simulink model "wind_pmsm_inv_dcBus"  (R2016a)
settings: Solver=VariableStepAuto  StartTime=0.0  StopTime=0.25*100e6  RelTol=1e-3
libraries: xbsIndex_r4 x34, powerlib_meascontrol x2
settings Model: Creator=Jorge  LastModifiedBy=Jorge

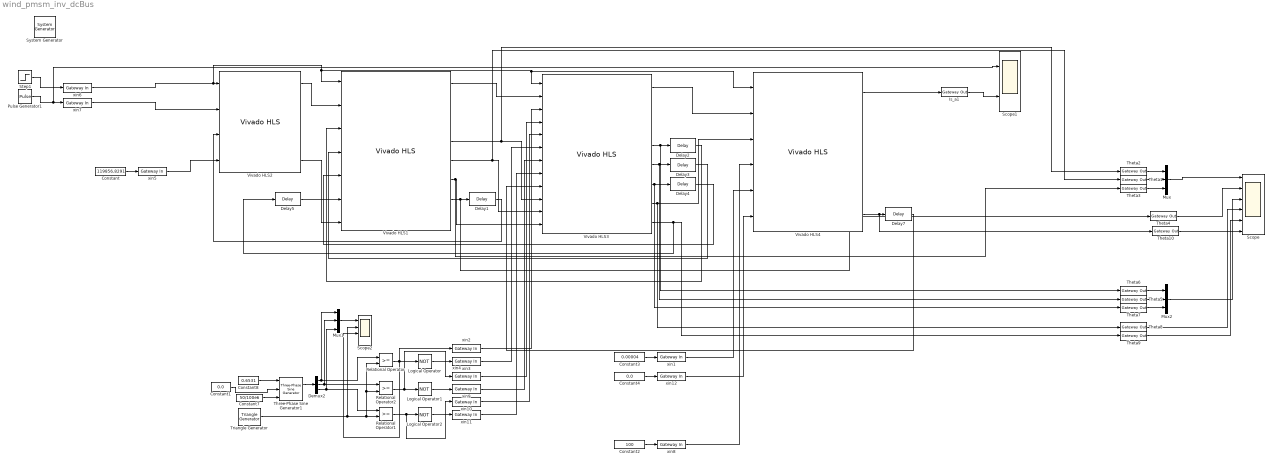
== system wind_pmsm_inv_dcBus ==
  " System Generator" : xbsIndex_r4/ System Generator  Tag=genX  xilinxfamily=zynq  part=xc7z020  speed=-1  package=clg400  synthesis_tool=Vivado  clock_wrapper=Clock Enables  directory=./netlist  proj_type=Vivado  Synth_file=Vivado Synthesis Defaults  Impl_file=Vivado Implementation Defaults  testbench=off  simulink_period=1  sysclk_period=10  dcm_input_clock_period=10  incr_netlist=off  trim_vbits=Everywhere in SubSystem  dbl_ovrd=According to Block Masks  core_generation=According to Block Masks  run_coregen=off  deprecated_control=off  eval_field=0  block_type=sysgen
  Constant : Constant  Value=119856.8291
  Constant1 : Constant  Value=0.0
  Constant2 : Constant  Value=100
  Constant3 : Constant  Value=0.00004
  Constant4 : Constant  Value=0.0
  Constant7 : Constant  Value=50/100e6
  Constant8 : Constant  Value=0.6531
  Delay{1..5,7} (6 alike) : xbsIndex_r4/Delay  rst=off  infoeditControl=Selection of Reset will increase slice count due to use of real FFs and instead of SRLs  en=off  latency=1  reg_retiming=off  dbl_ovrd=off  block_type=delay
  Demux2 : Demux  Outputs=3
  Is_a1 : xbsIndex_r4/Gateway Out  inherit_from_input=off  hdl_port=on  rows=1  columns=1  UseAsDAC=off  DACChannel='1'  interface=None  automatic_assignment=on  address_offset=hex2dec('00')  intf_name=''  intf_description=''  timing_constraint=None  locs_specified=off  LOCs={}  io_standard={}  block_type=gatewayout
  Logical Operator : Logic  Operator=NOT  AllPortsSameDT=off  OutDataTypeStr=boolean
  Logical Operator1 : Logic  Operator=NOT  AllPortsSameDT=off  OutDataTypeStr=boolean
  Logical Operator2 : Logic  Operator=NOT  AllPortsSameDT=off  OutDataTypeStr=boolean
  Mux : Mux  Inputs=3
  Mux1 : Mux  Inputs=3
  Mux2 : Mux  Inputs=3
  Pulse Generator1 : DiscretePulseGenerator  PulseType=Time based  Period=200
  Relational Operator : RelationalOperator  OutDataTypeStr=boolean  ZeroCross=off
  Relational Operator1 : RelationalOperator  OutDataTypeStr=boolean  ZeroCross=off
  Relational Operator2 : RelationalOperator  OutDataTypeStr=boolean  ZeroCross=off
  Scope : Scope  NumInputPorts=6
  Scope1 : Scope  NumInputPorts=2
  Scope2 : Scope  NumInputPorts=4
  Step1 : Step  Time=1e-6  SampleTime=0
  Theta{1..10} (10 alike) : xbsIndex_r4/Gateway Out  inherit_from_input=off  hdl_port=on  rows=1  columns=1  UseAsDAC=off  DACChannel='1'  interface=None  automatic_assignment=on  address_offset=hex2dec('00')  intf_name=''  intf_description=''  timing_constraint=None  locs_specified=off  LOCs={}  io_standard={}  block_type=gatewayout
  Three-Phase Sine Generator1 : powerlib_meascontrol/Pulse & Signal Generators/Three-Phase Sine Generator  Ts=1
  Triangle Generator : powerlib_meascontrol/Pulse & Signal Generators/Triangle Generator  Freq=5e3/100e6  Phase=0  Ts=1
  Vivado HLS1 : xbsIndex_r4/Vivado HLS  anytable='C:/Users/Jorge/Documents/GitHub/nvHIL/hls/pmsm_V2/pmsm_V2_prj/sol_sysgen'  fast_sim=off  display_datatype=on  rate_propagation_method=Simulink system period  model_file_path=''  latency=1  block_type=hls
      settings: infoedit=This block allows including C,C++ and SystemC source files in System Generator for DSP designs.
  Vivado HLS2 : xbsIndex_r4/Vivado HLS  anytable='C:\Users\Jorge\Documents\GitHub\nvHIL\hls\wind_tur_V2\wind_turb_V2_prj\sol_sysgen'  fast_sim=off  display_datatype=on  rate_propagation_method=Simulink system period  model_file_path=''  latency=1  block_type=hls
      settings: infoedit=This block allows including C,C++ and SystemC source files in System Generator for DSP designs.
  Vivado HLS3 : xbsIndex_r4/Vivado HLS  anytable='C:\Users\Jorge\Documents\GitHub\nvHIL\hls\pmsm_3ph_inv_V2\pmsm_inv_prj\sol_sysgen'  fast_sim=off  display_datatype=on  rate_propagation_method=Simulink system period  model_file_path=''  latency=1  block_type=hls
      settings: infoedit=This block allows including C,C++ and SystemC source files in System Generator for DSP designs.
  Vivado HLS4 : xbsIndex_r4/Vivado HLS  anytable='C:\Users\Jorge\Documents\GitHub\nvHIL\hls\DC_bus_V2\dc_bus_prj\sol_sysgen'  fast_sim=off  display_datatype=on  rate_propagation_method=Simulink system period  model_file_path=''  latency=1  block_type=hls
      settings: infoedit=This block allows including C,C++ and SystemC source files in System Generator for DSP designs.
  xin1 : xbsIndex_r4/Gateway In  gui_display_data_type=Fixed-point  arith_type="Signed  (2's comp)"  n_bits=19  bin_pt=18  preci_type=Single  exp_width=8  frac_width=24  rows=1  columns=1  quantization="Round  (unbiased: +/- Inf)"  overflow=Saturate  period=1  UseAsADC=off  ADCChannel='1'  interface=None  automatic_assignment=on  address_offset=hex2dec('00')  intf_name=''  intf_description=''  default_value=0  timing_constraint=None  locs_specified=off  LOCs={}  io_standard={}  inherit_from_input=off  hdl_port=on  dbl_ovrd=off  block_type=gatewayin
  xin{2..4,9..11} (6 alike) : xbsIndex_r4/Gateway In  gui_display_data_type=Boolean  arith_type=Boolean  n_bits=18  bin_pt=6  preci_type=Single  exp_width=8  frac_width=24  rows=1  columns=1  quantization="Round  (unbiased: +/- Inf)"  overflow=Saturate  period=1  UseAsADC=off  ADCChannel='1'  interface=None  automatic_assignment=on  address_offset=hex2dec('00')  intf_name=''  intf_description=''  default_value=0  timing_constraint=None  locs_specified=off  LOCs={}  io_standard={}  inherit_from_input=off  hdl_port=on  dbl_ovrd=off  block_type=gatewayin
  xin12 : xbsIndex_r4/Gateway In  gui_display_data_type=Fixed-point  arith_type="Signed  (2's comp)"  n_bits=2  bin_pt=1  preci_type=Single  exp_width=8  frac_width=24  rows=1  columns=1  quantization="Round  (unbiased: +/- Inf)"  overflow=Saturate  period=1  UseAsADC=off  ADCChannel='1'  interface=None  automatic_assignment=on  address_offset=hex2dec('00')  intf_name=''  intf_description=''  default_value=0  timing_constraint=None  locs_specified=off  LOCs={}  io_standard={}  inherit_from_input=off  hdl_port=on  dbl_ovrd=off  block_type=gatewayin
  xin5 : xbsIndex_r4/Gateway In  gui_display_data_type=Fixed-point  arith_type="Signed  (2's comp)"  n_bits=21  bin_pt=1  preci_type=Single  exp_width=8  frac_width=24  rows=1  columns=1  quantization="Round  (unbiased: +/- Inf)"  overflow=Saturate  period=1  UseAsADC=off  ADCChannel='1'  interface=None  automatic_assignment=on  address_offset=hex2dec('00')  intf_name=''  intf_description=''  default_value=0  timing_constraint=None  locs_specified=off  LOCs={}  io_standard={}  inherit_from_input=off  hdl_port=on  dbl_ovrd=off  block_type=gatewayin
  xin6 : xbsIndex_r4/Gateway In  gui_display_data_type=Boolean  arith_type=Boolean  n_bits=16  bin_pt=10  preci_type=Single  exp_width=8  frac_width=24  rows=1  columns=1  quantization="Round  (unbiased: +/- Inf)"  overflow=Saturate  period=1  UseAsADC=off  ADCChannel='1'  interface=None  automatic_assignment=on  address_offset=hex2dec('00')  intf_name=''  intf_description=''  default_value=0  timing_constraint=None  locs_specified=off  LOCs={}  io_standard={}  inherit_from_input=off  hdl_port=on  dbl_ovrd=off  block_type=gatewayin
  xin7 : xbsIndex_r4/Gateway In  gui_display_data_type=Boolean  arith_type=Boolean  n_bits=16  bin_pt=10  preci_type=Single  exp_width=8  frac_width=24  rows=1  columns=1  quantization="Round  (unbiased: +/- Inf)"  overflow=Saturate  period=1  UseAsADC=off  ADCChannel='1'  interface=None  automatic_assignment=on  address_offset=hex2dec('00')  intf_name=''  intf_description=''  default_value=0  timing_constraint=None  locs_specified=off  LOCs={}  io_standard={}  inherit_from_input=off  hdl_port=on  dbl_ovrd=off  block_type=gatewayin
  xin8 : xbsIndex_r4/Gateway In  gui_display_data_type=Fixed-point  arith_type="Signed  (2's comp)"  n_bits=25  bin_pt=9  preci_type=Single  exp_width=8  frac_width=24  rows=1  columns=1  quantization="Round  (unbiased: +/- Inf)"  overflow=Saturate  period=1  UseAsADC=off  ADCChannel='1'  interface=None  automatic_assignment=on  address_offset=hex2dec('00')  intf_name=''  intf_description=''  default_value=0  timing_constraint=None  locs_specified=off  LOCs={}  io_standard={}  inherit_from_input=off  hdl_port=on  dbl_ovrd=off  block_type=gatewayin
  wires:
  Step1/1 -> xin6/1
  Pulse Generator1/1 -> Scope1/1, xin7/1
  Is_a1/1 -> Scope1/2
  Constant/1 -> xin5/1
  Theta4/1 -> Scope/2
  xin6/1 -> Vivado HLS1/1, Vivado HLS3/1, Vivado HLS4/1, Vivado HLS2/1
  xin7/1 -> Vivado HLS2/2
  Vivado HLS2/1 -> Vivado HLS1/2
  Vivado HLS2/4 -> Vivado HLS1/7
  Delay1/1 -> Vivado HLS2/3
  xin5/1 -> Vivado HLS2/4
  Demux2/1 -> Mux1/1, Relational Operator/1
  Demux2/2 -> Mux1/2, Relational Operator2/1
  Demux2/3 -> Mux1/3, Relational Operator1/1
  Triangle Generator/1 -> Scope2/2, Relational Operator1/2, Relational Operator2/2, Relational Operator/2
  Relational Operator/1 -> xin2/1, Logical Operator/1, Scope2/3
  Constant7/1 -> Three-Phase Sine Generator1/3
  Constant8/1 -> Three-Phase Sine Generator1/1
  Three-Phase Sine Generator1/1 -> Demux2/1
  Mux1/1 -> Scope2/1
  Constant1/1 -> Three-Phase Sine Generator1/2
  Mux/1 -> Scope/1
  Theta2/1 -> Mux/1
  Theta1/1 -> Mux/2
  Theta3/1 -> Mux/3
  Vivado HLS1/7 -> Theta4/1, Delay1/1
  Vivado HLS1/1 -> Vivado HLS3/2
  Vivado HLS1/4 -> Theta2/1, Vivado HLS3/10
  Vivado HLS1/5 -> Theta1/1, Vivado HLS3/11
  Vivado HLS1/6 -> Theta3/1, Vivado HLS3/12
  Vivado HLS3/4 -> Theta6/1, Delay2/1
  Vivado HLS3/5 -> Theta5/1, Delay3/1
  Vivado HLS3/6 -> Theta7/1, Delay4/1
  Delay2/1 -> Vivado HLS1/3
  Delay3/1 -> Vivado HLS1/4
  Delay4/1 -> Vivado HLS1/5
  Theta6/1 -> Mux2/1
  Theta5/1 -> Mux2/2
  Theta7/1 -> Mux2/3
  Mux2/1 -> Scope/3
  Vivado HLS3/8 -> Delay5/1, Theta9/1
  Theta8/1 -> Scope/4
  Theta9/1 -> Scope/5
  Delay5/1 -> Vivado HLS1/6
  Relational Operator1/1 -> xin10/1, Logical Operator2/1
  Relational Operator2/1 -> xin4/1, Logical Operator1/1
  Logical Operator2/1 -> xin11/1
  Logical Operator1/1 -> xin9/1
  Logical Operator/1 -> xin3/1
  xin2/1 -> Vivado HLS3/3
  xin4/1 -> Vivado HLS3/4
  xin10/1 -> Vivado HLS3/5
  xin3/1 -> Vivado HLS3/6
  xin9/1 -> Vivado HLS3/7
  xin11/1 -> Vivado HLS3/8
  Vivado HLS3/1 -> Vivado HLS4/2
  Vivado HLS3/7 -> Vivado HLS4/3, Theta8/1
  Constant3/1 -> xin1/1
  xin1/1 -> Vivado HLS4/5
  Constant4/1 -> xin12/1
  xin12/1 -> Vivado HLS4/6
  Vivado HLS4/1 -> Is_a1/1
  Vivado HLS4/4 -> Theta10/1, Delay7/1
  Constant2/1 -> xin8/1
  xin8/1 -> Vivado HLS4/4
  Theta10/1 -> Scope/6
  Delay7/1 -> Vivado HLS3/9
